simulink model "FallProtectionsim_Final"  (R2022a)
settings: Solver=VariableStepAuto  StartTime=0.0  StopTime=3  RelTol=1e-3
values from neighbouring files (symbols this model uses):
  A = [0,-r/(2*J),0,0;k*r/2,0,-k/2,0;0,1/(2*m),0,0;0,0,1,0]    [FallProtection_Final.m]
  B = [1/J,0;0,0;0,1/m;0,0]    [FallProtection_Final.m]
  BTI = 0.005    [FallProtection_Final.m]
  C = eye(4)    [FallProtection_Final.m]
  D = zeros(4,2)    [FallProtection_Final.m]
  enc_count = 2000    [FallProtection_Final.m]
  g = 9.81    [FallProtection_Final.m]
  K = lqrd(A2,B2,Q,R,BTI)    [FallProtection_Final.m]
  k = 690    [FallProtection_Final.m]
  m = 1    [FallProtection_Final.m]
  N = 5.9    [FallProtection_Final.m]
  r = .05    (= 0.05)    [FallProtection_Final.m]
  Tmax = 1    [FallProtection_Final.m]
  v0 = -1.5    [FallProtection_Final.m]
  x0 = [v0/r,(bws)*2*m*g,v0,xi]    [FallProtection_Final.m]
  xi = .5    (= 0.5)    [FallProtection_Final.m]
undefined symbols (not defined in the file or in its folder): param
libraries: simulink x2, cstblocks x1, dspsrcs4 x1
settings Model: Creator=keita  LastModifiedBy=keita
settings DataIOCC: SaveFormat=Array

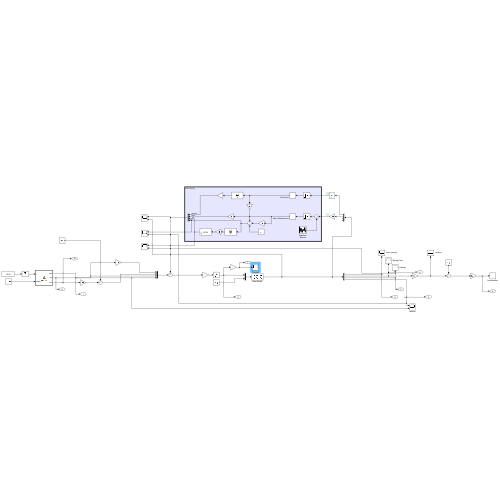
[thumbnail: Simulink's stored preview of the top-level diagram]
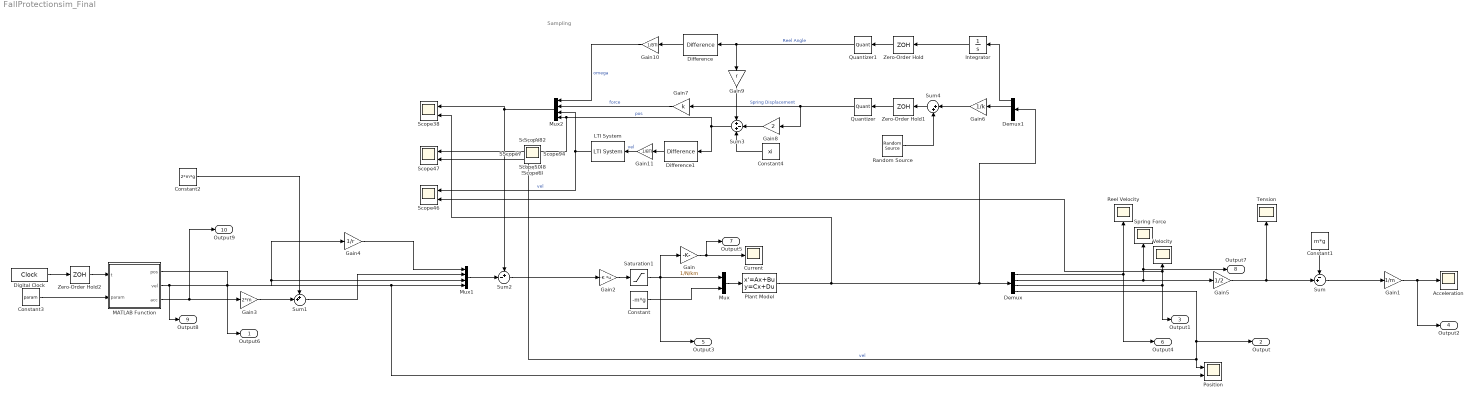
== system FallProtectionsim_Final ==
  note: Sampling
  Acceleration : Scope
  Constant : Constant  Value=-m*g
  Constant1 : Constant  Value=m*g
  Constant2 : Constant  Value=2*m*g
  Constant3 : Constant  Value=param
  Constant4 : Constant  Value=xi
  Current : Scope
  Demux : Demux
  Demux1 : Demux
  Difference : simulink/Discrete/Difference  ICPrevInput=0  OutMin=[]  OutMax=[]  OutDataType=fixdt(1, 16)  OutScaling=2^-10  DoSatur=off
  Difference1 : simulink/Discrete/Difference  ICPrevInput=xi-v0*BTI  OutMin=[]  OutMax=[]  OutDataType=fixdt(1, 16)  OutScaling=2^-10  DoSatur=off
  Digital Clock : DigitalClock  SampleTime=.005
  Gain : Gain  Gain=1/N/km
  Gain1 : Gain  Gain=1/m
  Gain10 : Gain  Gain=1/BTI
  Gain11 : Gain  Gain=1/BTI
  Gain2 : Gain  Gain=-K  Multiplication=Matrix(K*u)
  Gain3 : Gain  Gain=2*m
  Gain4 : Gain  Gain=1/r
  Gain5 : Gain  Gain=1/2
  Gain6 : Gain  Gain=1/k
  Gain7 : Gain  Gain=k
  Gain8 : Gain  Gain=2
  Gain9 : Gain  Gain=r
  Integrator : Integrator
  LTI System : cstblocks/LTI System  sys=LPFd  IC=[]
  MATLAB Function : MATLAB Function  TreatAsAtomicUnit=on
  Mux : Mux  Inputs=2
  Mux1 : Mux
  Mux2 : Mux
  Plant Model : StateSpace  A=A  B=B  C=C  D=D  InitialCondition=x0
  Position : Scope  NumInputPorts=2
  Quantizer : Quantizer  QuantizationInterval=.1/2^12
  Quantizer1 : Quantizer  QuantizationInterval=2*pi/enc_count/N
  Random Source : dspsrcs4/Random Source  SrcType=Gaussian  NormMethod=Ziggurat  CltLength=12  MinVal=0  MaxVal=1  MeanVal=0  VarVal=3.8e-11  RepMode=Not repeatable  rawSeed=1  IsInherit=off  SampMode=Continuous  SampTime=BTI  SampFrame=1  DataType=Single  OutComplex=Real  OutputFrames=off
  Reel Velocity : Scope
  Saturation1 : Saturate  UpperLimit=Tmax  LowerLimit=-Tmax
  Scope38 : Scope  NumInputPorts=2
  Scope46 : Scope  NumInputPorts=2
  Scope47 : Scope  NumInputPorts=2
  Spring Force : Scope
  Sum : Sum  Inputs=-+|
  Sum1 : Sum  Inputs=++|
  Sum2 : Sum  Inputs=+-|
  Sum3 : Sum  Inputs=+-+
  Sum4 : Sum  Inputs=|++
  Tension : Scope
  Velocity : Scope
  Zero-Order Hold : ZeroOrderHold  SampleTime=BTI
  Zero-Order Hold1 : ZeroOrderHold  SampleTime=BTI
  Zero-Order Hold2 : ZeroOrderHold  SampleTime=BTI
  Output6 : Outport
  Output : Outport  Port=2
  Output1 : Outport  Port=3
  Output2 : Outport  Port=4
  Output3 : Outport  Port=5
  Output4 : Outport  Port=6
  Output5 : Outport  Port=7
  Output7 : Outport  Port=8
  Output8 : Outport  Port=9
  Output9 : Outport  Port=10
  Scope{,1..37,39..45,48..50} (48 alike) : Scope
  wires:
  Constant/1 -> Mux/2
  Constant3/1 -> MATLAB Function/2(param)
  Demux/1 -> Reel Velocity/1, Output4/1
  Mux/1 -> Plant Model/1
  Mux1/1 -> Sum2/2
  MATLAB Function/1(pos) -> Position/2, Mux1/4, Output6/1
  Gain/1 -> Output5/1, Current/1
  Gain5/1 -> Sum/2, Tension/1
  Constant1/1 -> Sum/1
  Sum/1 -> Gain1/1
  Gain1/1 -> Output2/1, Acceleration/1
  Demux/3 -> Output1/1, Scope46/2, Velocity/1
  Sum1/1 -> Mux1/2
  Sum2/1 -> Gain2/1
  Gain4/1 -> Mux1/1
  Constant2/1 -> Sum1/1
  MATLAB Function/3(acc) -> Output9/1, Gain3/1
  Gain3/1 -> Sum1/2
  MATLAB Function/2(vel) -> Gain4/1, Mux1/3, Output8/1
  Demux/2 -> Gain5/1, Spring Force/1, Output7/1
  Demux1/2 -> Gain6/1
  Gain7/1 -> Mux2/2  "force"
  Gain10/1 -> Mux2/1  "omega"
  Sum3/1 -> Difference1/1, Scope47/1, Mux2/4  "pos"
  Gain8/1 -> Sum3/2
  Difference1/1 -> Gain11/1
  Gain9/1 -> Sum3/1
  Constant4/1 -> Sum3/3
  Gain2/1 -> Saturation1/1
  Quantizer1/1 -> Difference/1, Gain9/1  "Reel Angle"
  Quantizer/1 -> Gain8/1, Gain7/1  "Spring Displacement"
  Gain6/1 -> Sum4/1
  Saturation1/1 -> Gain/1, Output3/1, Mux/1
  Demux/4 -> Output/1, Scope47/2, Position/1  "vel"
  Random Source/1 -> Sum4/2
  Sum4/1 -> Zero-Order Hold1/1
  Difference/1 -> Gain10/1
  LTI System/1 -> Mux2/3, Scope46/1  "vel"
  Plant Model/1 -> Scope38/2, Demux1/1, Demux/1
  Digital Clock/1 -> Zero-Order Hold2/1
  Mux2/1 -> Sum2/1, Scope38/1
  Zero-Order Hold/1 -> Quantizer1/1
  Zero-Order Hold1/1 -> Quantizer/1
  Zero-Order Hold2/1 -> MATLAB Function/1(t)
  Demux1/1 -> Integrator/1
  Integrator/1 -> Zero-Order Hold/1
  Gain11/1 -> LTI System/1  "vel"

== matlab function FallProtectionsim_Final/MATLAB Function ==
  settings: updateMethod=DISCRETE
  data: t input; pos output; param input; vel output; acc output
function [pos,vel,acc] = sramp(t,param)
xi = param(1);
xf = param(2);
v0 = param(3);
vmax = param(4);
amax = param(5);

totalDist = xf-xi;
accTime = (vmax-v0)/amax;
accDist = v0*accTime+1/2*amax*accTime^2;

decelTime = vmax/amax;
decelDist = 1/2*amax*decelTime^2;

if (totalDist<=accDist+decelDist)
        % No constant velocity phase
        decelTime = sqrt((totalDist+(v0^2/(2*amax)))/amax);
        accTime = decelTime-v0/amax;
        totalTime = accTime+decelTime;
        velTime = 0;
        velDist = 0;
        vmax = 0;
    else
        % With constant velocity phase
        velDist = totalDist-accDist-decelDist;
        velTime = velDist/vmax;
        totalTime = accTime+decelTime+velTime;
end

if t<accTime
    pos = xi+v0*t+1/2*amax*t^2;
    vel = v0+amax*t;
    acc = amax;
elseif t>=accTime && t<(accTime+velTime)
    pos = xi+accDist+vmax*(t-accTime);
    vel = vmax;
    acc = 0;
elseif t>=(accTime+velTime) && t<totalTime
    pos = xf-1/2*amax*(totalTime-t)^2;
    vel = amax*(totalTime-t);
    acc = -amax;
else
    pos = xf;
    vel = 0;
    acc = 0;
end
end
